simulink model "entryVehicle"  (R2024b)
settings: Solver=ode5  StartTime=startTime  StopTime=stopTime  FixedStep=stepTime  RelTol=1e-3
values from neighbouring files (symbols this model uses):
  acce_bias = [0; 0; 0]    [run_entryVehicle.m]
  acce_S = [0, 0, 0 ... (first row only)    [run_entryVehicle.m]
  alpha_0 = deg2rad(-23.82)    [run_entryVehicle.m]
  beta_0 = deg2rad(0.0)    [run_entryVehicle.m]
  chi_0 = deg2rad(90)    [run_entryVehicle.m]
  d_ref = 3.9    [run_entryVehicle.m]
  gamma_0 = deg2rad(-9.536)    [run_entryVehicle.m]
  H_s = 7050    [run_entryVehicle.m]
  I_xx = 5617.61    [run_entryVehicle.m]
  I_xz = 0    [run_entryVehicle.m]
  I_yy = 4454.62    [run_entryVehicle.m]
  I_zz = 4454.80    (= 4454.8)    [run_entryVehicle.m]
  lambda_0 = deg2rad(0)    [run_entryVehicle.m]
  m_0 = 4976    [run_entryVehicle.m]
  Mars_radius = 6371e3    (= 6371000)    [run_entryVehicle.m]
  p_0 = deg2rad(0)    [run_entryVehicle.m]
  Q0 = [Q1; Q2; Q3; Q4]    [get_Q0.m]    (also in run_entryVehicle.m = get_Q0(tau_0, lambda_0, chi_0, gamma_0, alpha_0, beta_0, sig)
  q_0 = deg2rad(0)    [run_entryVehicle.m]
  r0_eci = [x; y; z]    [getInitialECI.m]
  r_0 = deg2rad(0)    [run_entryVehicle.m]
  R_0 = 220e3 + Mars_radius    (= 6591000)    [run_entryVehicle.m]
  r_cm = [-0.137; 0; 1.8]    [run_entryVehicle.m]
  R_s = 287    [run_entryVehicle.m]
  rateGyro_bias = [0; 0; 0]    [run_entryVehicle.m]
  rateGyro_S = [0, 0, 0 ... (first row only)    [run_entryVehicle.m]
  rho_0 = 1.225    [run_entryVehicle.m]
  S_ref = 12    [run_entryVehicle.m]
  sigma_0 = deg2rad(100.)    [run_entryVehicle.m]
  specific_heat = 1.29    [run_entryVehicle.m]
  stepTime = 0.01    [run_entryVehicle.m]
  tau_0 = deg2rad(0)    [run_entryVehicle.m]
  v0_eci = T_ECI_NED * v_ned    [getInitialECI.m]
  V_0 = 11e3    (= 11000)    [run_entryVehicle.m]
undefined symbols (not defined in the file or in its folder): A_attitude, alpha_T_CD, alpha_T_CL, alpha_T_Cm, alpha_T_Cm_q, B_attitude, CD_T, CL_T, Cm_qT, Cm_T, K_lat, K_long, lateral_ref, longitudinal_ref, Mach_numbers_CD, Mach_numbers_CL, Mach_numbers_Cm, Mach_numbers_Cm_q, Mars_mu, my_max
libraries: simulink_extras x33, aerolibnav x2, simulink x1, SignalEditorBlockLib x1
(part 2 of 2)

== system entryVehicle/State Space/References ==
  lateral_ref : Constant  Value=lateral_ref
  longitudinal_ref : Constant  Value=longitudinal_ref
  out_longitudinal ref : Outport
  out_lateral_ref : Outport  Port=2
  wires:
  longitudinal_ref/1 -> out_longitudinal ref/1
  lateral_ref/1 -> out_lateral_ref/1

== system entryVehicle/Plant/Atmosphere/Atmospheric Density ==
  h : Inport
  Constant : Constant  Value=rho_0  SampleTime=stepTime
  Constant1 : Constant  Value=H_s  SampleTime=stepTime
  MATLAB Function : MATLAB Function  TreatAsAtomicUnit=on
  rho : Outport
  wires:
  h/1 -> MATLAB Function/1(h)
  Constant1/1 -> MATLAB Function/3(H_s)
  Constant/1 -> MATLAB Function/2(rho_0)
  MATLAB Function/1(rho) -> rho/1

== system entryVehicle/Plant/Dynamics/Attitude Dynamics ==
  M_x : Inport
  M_y : Inport  Port=2
  M_z : Inport  Port=3
  p : Inport  Port=4
  q : Inport  Port=5
  r : Inport  Port=6
  Ixx : Inport  Port=7
  Iyy : Inport  Port=8
  Izz : Inport  Port=9
  Ixz : Inport  Port=10
  Integrator : Integrator  InitialCondition=p_0
  Integrator1 : Integrator  InitialCondition=q_0
  Integrator2 : Integrator  InitialCondition=r_0
  MATLAB Function1 : MATLAB Function  TreatAsAtomicUnit=on
  Mux : Mux  Inputs=3
  p,q,r : Outport
  wires:
  MATLAB Function1/2(q_dot) -> Integrator1/1
  MATLAB Function1/1(p_dot) -> Integrator/1
  MATLAB Function1/3(r_dot) -> Integrator2/1
  Integrator/1 -> Mux/1  "p"
  Integrator1/1 -> Mux/2  "q"
  Integrator2/1 -> Mux/3  "r"
  Mux/1 -> p,q,r/1
  M_x/1 -> MATLAB Function1/1(M_x)
  M_y/1 -> MATLAB Function1/2(M_y)
  M_z/1 -> MATLAB Function1/3(M_z)
  p/1 -> MATLAB Function1/4(p)
  q/1 -> MATLAB Function1/5(q)
  r/1 -> MATLAB Function1/6(r)
  Ixx/1 -> MATLAB Function1/7(Ixx)
  Iyy/1 -> MATLAB Function1/8(Iyy)
  Izz/1 -> MATLAB Function1/9(Izz)
  Ixz/1 -> MATLAB Function1/10(Ixz)

== system entryVehicle/Plant/Dynamics/Heat_Flux ==
  rho : Inport
  V : Inport  Port=2
  MATLAB Function : MATLAB Function  TreatAsAtomicUnit=on
  To Workspace : ToWorkspace  VariableName=q_c  SaveFormat=Timeseries  SampleTime=-1
  q_c : Outport
  wires:
  rho/1 -> MATLAB Function/2(rho)
  V/1 -> MATLAB Function/1(V)
  MATLAB Function/1(q_c) -> To Workspace/1, q_c/1

== system entryVehicle/Plant/Dynamics/Translation Dynamics ==
  D : Inport
  L : Inport  Port=2
  S : Inport  Port=3
  V : Inport  Port=4
  gamma : Inport  Port=5
  chi : Inport  Port=6
  sigma : Inport  Port=7
  R : Inport  Port=8
  lambda : Inport  Port=9
  m : Inport  Port=10
  g : Inport  Port=11
  Integrator : Integrator  InitialCondition=V_0
  Integrator1 : Integrator  InitialCondition=gamma_0
  Integrator2 : Integrator  InitialCondition=chi_0
  MATLAB Function : MATLAB Function  TreatAsAtomicUnit=on
  Mux : Mux  Inputs=3
  V,gamma,chi : Outport
  wires:
  MATLAB Function/1(V_dot) -> Integrator/1
  MATLAB Function/2(gamma_dot) -> Integrator1/1
  MATLAB Function/3(chi_dot) -> Integrator2/1
  Integrator/1 -> Mux/1  "V"
  Integrator1/1 -> Mux/2  "gamma"
  Integrator2/1 -> Mux/3  "chi"
  Mux/1 -> V,gamma,chi/1
  D/1 -> MATLAB Function/1(D)
  L/1 -> MATLAB Function/2(L)
  S/1 -> MATLAB Function/3(S)
  V/1 -> MATLAB Function/4(V)
  gamma/1 -> MATLAB Function/5(gamma)
  chi/1 -> MATLAB Function/6(chi)
  sigma/1 -> MATLAB Function/7(sigma)
  R/1 -> MATLAB Function/8(R)
  lambda/1 -> MATLAB Function/9(lambda)
  m/1 -> MATLAB Function/10(m)
  g/1 -> MATLAB Function/11(g)

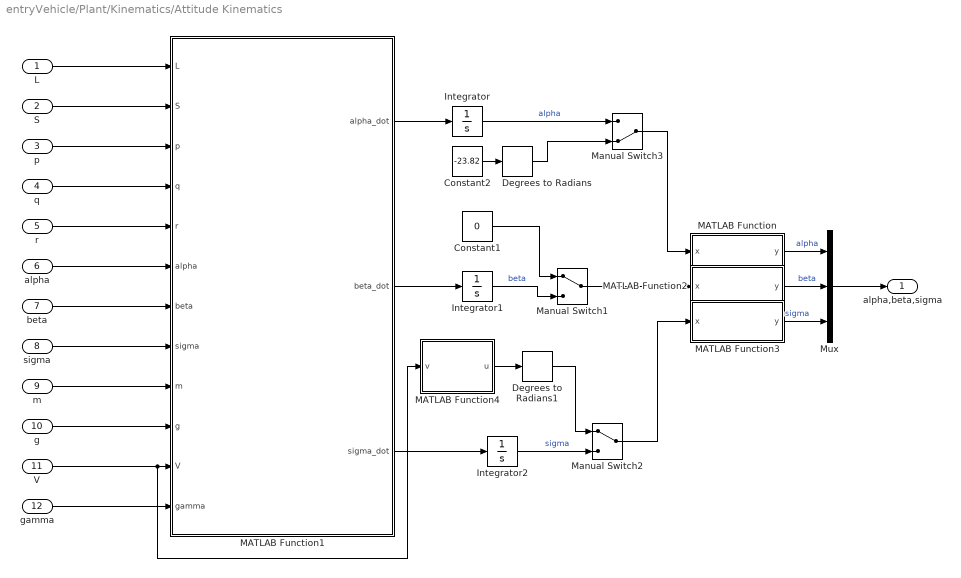
== system entryVehicle/Plant/Kinematics/Attitude Kinematics ==
  L : Inport
  S : Inport  Port=2
  p : Inport  Port=3
  q : Inport  Port=4
  r : Inport  Port=5
  alpha : Inport  Port=6
  beta : Inport  Port=7
  sigma : Inport  Port=8
  m : Inport  Port=9
  g : Inport  Port=10
  V : Inport  Port=11
  gamma : Inport  Port=12
  Constant1 : Constant  Value=0
  Constant2 : Constant  Value=-23.82
  Degrees to Radians : simulink_extras/Transformations/Degrees to Radians
  Degrees to Radians1 : simulink_extras/Transformations/Degrees to Radians
  Integrator : Integrator  InitialCondition=alpha_0
  Integrator1 : Integrator  InitialCondition=beta_0
  Integrator2 : Integrator  InitialCondition=sigma_0
  MATLAB Function : MATLAB Function  TreatAsAtomicUnit=on
  MATLAB Function1 : MATLAB Function  TreatAsAtomicUnit=on
  MATLAB Function2 : MATLAB Function  TreatAsAtomicUnit=on
  MATLAB Function3 : MATLAB Function  TreatAsAtomicUnit=on
  MATLAB Function4 : MATLAB Function  TreatAsAtomicUnit=on
  Manual Switch1 : ManualSwitch
  Manual Switch2 : ManualSwitch
  Manual Switch3 : ManualSwitch  CurrentSetting=0
  Mux : Mux  Inputs=3
  alpha,beta,sigma : Outport
  wires:
  beta/1 -> MATLAB Function1/7(beta)
  q/1 -> MATLAB Function1/4(q)
  m/1 -> MATLAB Function1/9(m)
  p/1 -> MATLAB Function1/3(p)
  sigma/1 -> MATLAB Function1/8(sigma)
  alpha/1 -> MATLAB Function1/6(alpha)
  L/1 -> MATLAB Function1/1(L)
  r/1 -> MATLAB Function1/5(r)
  g/1 -> MATLAB Function1/10(g)
  V/1 -> MATLAB Function4/1(v), MATLAB Function1/11(V)
  Mux/1 -> alpha,beta,sigma/1
  gamma/1 -> MATLAB Function1/12(gamma)
  MATLAB Function/1(y) -> Mux/1  "alpha"
  MATLAB Function2/1(y) -> Mux/2  "beta"
  MATLAB Function3/1(y) -> Mux/3  "sigma"
  S/1 -> MATLAB Function1/2(S)
  MATLAB Function1/1(alpha_dot) -> Integrator/1
  MATLAB Function1/2(beta_dot) -> Integrator1/1
  MATLAB Function1/3(sigma_dot) -> Integrator2/1
  Constant2/1 -> Degrees to Radians/1
  Integrator/1 -> Manual Switch3/1  "alpha"
  Manual Switch3/1 -> MATLAB Function/1(x)
  Manual Switch1/1 -> MATLAB Function2/1(x)
  Integrator1/1 -> Manual Switch1/2  "beta"
  Constant1/1 -> Manual Switch1/1
  Manual Switch2/1 -> MATLAB Function3/1(x)
  Integrator2/1 -> Manual Switch2/2  "sigma"
  Degrees to Radians/1 -> Manual Switch3/2
  Degrees to Radians1/1 -> Manual Switch2/1
  MATLAB Function4/1(u) -> Degrees to Radians1/1

== system entryVehicle/Plant/Kinematics/Translation Kinematics ==
  V : Inport
  gamma : Inport  Port=2
  chi : Inport  Port=3
  R : Inport  Port=4
  lambda : Inport  Port=5
  Integrator : Integrator  InitialCondition=R_0
  Integrator1 : Integrator  InitialCondition=tau_0
  Integrator2 : Integrator  InitialCondition=lambda_0
  MATLAB Function : MATLAB Function  TreatAsAtomicUnit=on
  Mux : Mux  Inputs=3
  R,tau,lambda : Outport
  wires:
  V/1 -> MATLAB Function/1(V)
  gamma/1 -> MATLAB Function/2(gamma)
  chi/1 -> MATLAB Function/3(chi)
  R/1 -> MATLAB Function/4(R)
  lambda/1 -> MATLAB Function/5(lambda)
  MATLAB Function/1(R_dot) -> Integrator/1
  MATLAB Function/2(tau_dot) -> Integrator1/1
  MATLAB Function/3(lambda_dot) -> Integrator2/1
  Integrator/1 -> Mux/1
  Integrator1/1 -> Mux/2
  Integrator2/1 -> Mux/3
  Mux/1 -> R,tau,lambda/1

== matlab function entryVehicle/Plant/Dynamics/Translation Dynamics/MATLAB Function ==
  data: V_dot output; gamma_dot output; chi_dot output; D input; L input; S input; V input; gamma input; chi input; sigma input; R input; lambda input; m input; g input
function [V_dot, gamma_dot, chi_dot] = Translation_Dynamics(D, L, S, V, gamma, chi, sigma, R, lambda, m, g)

V_dot = -D/m - g*sin(gamma);
gamma_dot = (V/R - g/V)*cos(gamma) + (L*cos(sigma) - S*sin(sigma))/(m*V);
chi_dot = V/R*cos(gamma)*tan(lambda)*sin(chi) - (L*sin(sigma) + S*cos(sigma))/(m*V*cos(gamma));

== matlab function entryVehicle/Plant/Aerodynamic Data (Apex reference frame)/MATLAB Function1 ==
  data: alpha input; alphaT output; beta input
function alphaT = total_angleAttack(alpha, beta)

alphaT = acos(cos(alpha)*cos(beta));

== matlab function entryVehicle/Plant/Aerodynamic Data (Apex reference frame)/MATLAB Function2 ==
  data: C_m output; C_mT input; C_n output; alpha input; beta input; alphaT input
function [C_m, C_n] = CmTtransformation(C_mT, alpha, beta, alphaT)

epsilon = 1e-6; % Threshold to detect near-zero total angle

if abs(alphaT) < epsilon
    % At singularity: alpha = beta = 0, so just return total coefficient for pitch moment, no yaw moment
    C_m = C_mT;
    C_n = 0;
else
    % Regular transformation
    C_m = sin(alpha)*cos(beta)/sin(alphaT) * C_mT;
    C_n = -sin(beta)/sin(alphaT) * C_mT;
end

== matlab function entryVehicle/Plant/Aerodynamic Data (Apex reference frame)/MATLAB Function3 ==
  data: C_mq output; C_mqT input; C_nr output; alpha input; beta input; alphaT input
function [C_mq, C_nr] = CmqTtransformation(C_mqT, alpha, beta, alphaT)

epsilon = 1e-6; % Threshold to detect near-zero total angle

if abs(alphaT) < epsilon
    % At singularity: alpha = beta = 0, so just return total coefficient for pitch moment, no yaw moment
    C_mq = C_mqT;
    C_nr = 0;
else
    % Regular transformation
    C_mq = sin(alpha)*cos(beta)/sin(alphaT) * C_mqT;
    C_nr = -sin(beta)/sin(alphaT) * C_mqT;
end

== matlab function entryVehicle/Plant/Kinematics/Attitude Kinematics/MATLAB Function ==
  data: x input; y output
function y = wrap_angle(x)
    y = wrapToPi(x);
end

== matlab function entryVehicle/Plant/Kinematics/Attitude Kinematics/MATLAB Function2 ==
  data: x input; y output
function y = wrap_angle(x)
    y = wrapToPi(x);
end

== matlab function entryVehicle/Plant/Kinematics/Attitude Kinematics/MATLAB Function3 ==
  data: x input; y output
function y = wrap_angle(x)
    y = wrapToPi(x);
end

== matlab function entryVehicle/Plant/Moments/MATLAB Function ==
  data: Mx_cross output; My_cross output; Mz_cross output; X_A input; Y_A input; Z_A input; r_cm input
function [Mx_cross, My_cross, Mz_cross] = crossProduct(X_A, Y_A, Z_A, r_cm)
    % Force vector in apex axes: [X; Y; Z]
    F_A_apex = [X_A; Y_A; Z_A];

    % Cross product to shift moment from apex to center of mass
    M_cross = cross(r_cm, F_A_apex);

    % Output individual components
    Mx_cross = M_cross(1);
    My_cross = M_cross(2);
    Mz_cross = M_cross(3);
end

== matlab function entryVehicle/Plant/Moments/MATLAB Function1 ==
  data: D input; X_A output; L input; S input; alpha input; beta input; Y_A output; Z_A output
function [X_A, Y_A, Z_A] = aeroFrame2apexFrameForces(D, L, S, alpha, beta)

c_alpha = cos(alpha);
s_alpha = sin(alpha);
c_beta = cos(beta);
s_beta = sin(beta);

X_A = -D*c_alpha*c_beta + S*c_alpha*s_beta + L*s_alpha;
Y_A = -D*s_beta - S*c_beta;
Z_A = -D*s_alpha*c_beta + S*s_alpha*s_beta - L*c_alpha;

== matlab function entryVehicle/State Space/MATLAB Function ==
  data: My input; u output; Mtx_Mtz input
function u = combine(My, Mtx_Mtz)
    Mx = Mtx_Mtz(1);
    Mz = Mtx_Mtz(2);
    
    u = [Mx; My; Mz];
end

== matlab function entryVehicle/Controller/Lateral Gain Scheduling/MATLAB Function ==
  data: Mach input; K_lat output
function K_lat = getLateralGain(Mach)
%#codegen
persistent Mach_Klat K_lat_data

if isempty(Mach_Klat)
    S = load('KLateralLUT.mat');  % Loads [N x 8]
    Mach_Klat = S.Mach_Klat;
    K_lat_data = S.K_lat_data;  % N x 8 (flattened 2x4)
end

% Interpolate 8 gains
K_lat_flat = interp1(Mach_Klat, K_lat_data, Mach, 'linear', 'extrap');

% Reshape into 2x4 matrix
K_lat = reshape(K_lat_flat, [2, 4]);
end

== matlab function entryVehicle/Controller/Longitude Gain Scheduling/MATLAB Function ==
  data: Mach input; K_long output
function K_long = getLongitudinalGain(Mach)
%#codegen
persistent Mach_Klong K_long_data

if isempty(Mach_Klong)
    S = load('KLongitudinalLUT.mat');  % <-- Load into struct first
    Mach_Klong = S.Mach_Klong;
    K_long_data = S.K_long_data;
end

% Interpolate both gains
K_long1 = interp1(Mach_Klong, K_long_data, Mach, 'linear', 'extrap');  % returns 1x2 vector
K_long = K_long1.';  % Now it's [2x1]
end

== matlab function entryVehicle/Controller/Integrator Subsystem/MATLAB Function ==
  data: Mach input; K_integrator_sigma output
function K_integrator_sigma = getIntsigmaGain(Mach)
%#codegen
persistent Mach_Ksigma K_sigmaInt_data

if isempty(Mach_Ksigma)
    S = load('KsigmaIntLUT.mat');  % Loads gain schedule
    Mach_Ksigma = S.Mach_Ksigma;          % Breakpoints
    K_sigmaInt_data = S.K_sigmaInt_data;  % Scalar gains
end

% Interpolate scalar gain based on Mach
K_integrator_sigma = interp1(Mach_Ksigma, K_sigmaInt_data, Mach, 'linear', 'extrap');
end

== matlab function entryVehicle/Controller/Integrator Subsystem1/MATLAB Function ==
  data: Mach input; K_integrator_alpha output
function K_integrator_alpha= getIntalphaGain(Mach)
%#codegen
persistent Mach_Ksigma K_sigmaInt_data

if isempty(Mach_Ksigma)
    S = load('KsigmaIntLUT.mat');  % Loads gain schedule
    Mach_Ksigma = S.Mach_Ksigma;          % Breakpoints
    K_sigmaInt_data = S.K_sigmaInt_data;  % Scalar gains
end

% Interpolate scalar gain based on Mach
K_integrator_alpha = interp1(Mach_Ksigma, K_sigmaInt_data, Mach, 'linear', 'extrap');
end

== matlab function entryVehicle/Plant/Kinematics/Attitude Kinematics/MATLAB Function4 ==
  data: v input; u output
function u = reference(v)

if v >= 3500
    u = 100;
elseif v <= 1500
    u = 75;
else
    u = 75 + (100 - 75) * (v - 1500) / (3500 - 1500);
end

== matlab function entryVehicle/Plant/Dynamics/Heat_Flux/MATLAB Function ==
  data: V input; q_c output; rho input
function q_c = heatFluxChapman(V, rho)
%#codegen

% Constants
c1 = 1.83e-4;     % empirical constant [SI]
c2 = 3.0;   % velocity exponent
d_ref = 3.9;
Rn = d_ref;         % nose radius [m]

% Chapman cold-wall heat flux equation
q_c = c1 / sqrt(Rn) * sqrt(rho) * V^c2;
end

== matlab function entryVehicle/Navigation/IMU Sensor2/MATLAB Function ==
  data: g_vec output; r input
function g_vec = computegvec(r)
% r    : 3x1 position vector in ECI frame (m)
% Constants
mu = 3.98319648e14; % Earth's gravitational parameter (m^3/s^2)

% Compute gravity vector in inertial frame
r_norm = norm(r);
g_vec1 = -mu / r_norm^3 * r;
g_vec=g_vec1';
end

== matlab function entryVehicle/Guidance/MATLAB Function ==
  data: x input; h output; s_dot output; m input; S_ref input; beta input; L_D input; rho_0 input; H_s input; v_dot output; L_D output; m output; gamma_dot output; h_dot output; D output
function [h,s_dot, v_dot, L_D, m, gamma_dot, h_dot, D] = entry_dynamics_derivatives(x, m, S_ref, beta, L_D, rho_0, H_s)
% Computes simplified translational dynamics for entry guidance
%
% Inputs:
%   x      : state vector [R; tau; delta; alpha; beta; sigma; v; gamma; chi; p; q; r]
%   m      : vehicle mass [kg]
%   S_ref  : reference area [m^2]
%   beta   : ballistic coefficient [kg/m^2]
%   L_D    : lift-to-drag ratio
%   rho_0  : reference atmospheric density [kg/m^3]
%   H_s    : scale height of the atmosphere [m]
%
% Output:
%   x_dot  : [s_dot; v_dot; gamma_dot; h_dot]

% ==== 1. Unpack necessary state variables ====
Mars_radius = 6371e3;
R     = x(1);   % Radius [m]
h = R-Mars_radius;
sigma = x(6);   % Bank angle [rad]
v     = x(7);   % Velocity [m/s]
gamma = x(8);   % Flight path angle [rad]

% ==== 2. Constants ====
Re = 6371e3;         % Earth radius [m]
g0 = 9.80665;        % Gravity at sea level [m/s^2]
h  = R - Re;         % Altitude [m]
gs = g0 * (Re / R)^2;  % Local gravity at R

% ==== 3. Atmospheric density ====
rho = rho_0 * exp(-h / H_s);

% ==== 4. Drag and Lift ====
C_D = m / (beta * S_ref);                      % Drag coefficient
D   = 0.5 * rho * v^2 * C_D * S_ref;           % Drag force [N]
L   = L_D * D;                                 % Lift force [N]

% ==== 5. Equations ====
s_dot     = v * cos(gamma);                                % Range rate
v_dot     = - (D/m + gs * sin(gamma));                     % Velocity rate
gamma_dot = (L * cos(sigma)) / (m * v) + ...
            ((v / R) - (gs / v)) * cos(gamma);             % Flight path angle rate
h_dot     = v * sin(gamma);                                % Altitude rate
end

== matlab function entryVehicle/Navigation/IMU Sensor3/MATLAB Function ==
  data: g_vec output; r input
function g_vec = computegvec(r)
% r    : 3x1 position vector in ECI frame (m)
% Constants
mu = 3.98319648e14; % Earth's gravitational parameter (m^3/s^2)

% Compute gravity vector in inertial frame
r_norm = norm(r);
g_vec1 = -mu / r_norm^3 * r;
g_vec=g_vec1';
end

== matlab function entryVehicle/Navigation/IMU Sensor3/MATLAB Function6 ==
  data: Q input; omega input; Q_dot output
function Q_dot = quat_kinematics(Q, omega)
    % omega: 3x1 vector [wx; wy; wz]
    % Q: 4x1 quaternion [q1; q2; q3; q4] (q4 is scalar part)
    Omega = [     0   -omega(1) -omega(2) -omega(3);
               omega(1)     0    omega(3) -omega(2);
               omega(2) -omega(3)     0    omega(1);
               omega(3)  omega(2) -omega(1)     0   ];
    Q_dot = 0.5 * Omega * Q;
end

== matlab function entryVehicle/Navigation/IMU Sensor3/MATLAB Function7 ==
  data: Q input; TIC output
function TIC = quatToDCM(Q)
% Q = [q1; q2; q3; q4]  (q4 is scalar part)

q1 = Q(1); q2 = Q(2); q3 = Q(3); q4 = Q(4);
TIC = [1 - 2*(q2^2 + q3^2),     2*(q1*q2 + q3*q4),     2*(q1*q3 - q2*q4);
     2*(q1*q2 - q3*q4),       1 - 2*(q1^2 + q3^2),   2*(q2*q3 + q1*q4);
     2*(q1*q3 + q2*q4),       2*(q2*q3 - q1*q4),     1 - 2*(q1^2 + q2^2)];
end

== matlab function entryVehicle/Navigation/State to Body (acce minus gravity)/MATLAB Function3 ==
  data: alpha_beta_sigma input; V_gamma_chi input; g_b output; R_tau_delta input; mu input
function g_b = computeGravityBody(alpha_beta_sigma, V_gamma_chi, R_tau_delta, mu)
    
    alpha = alpha_beta_sigma(1);
    beta = alpha_beta_sigma(2);
    sigma = alpha_beta_sigma(3);

    gamma = V_gamma_chi(2);
    chi = V_gamma_chi(3);

    R = R_tau_delta(1);

    % Gravity in vertical frame (downward)
    g_v = [0; 0; mu / R^2];

    % Precompute trigonometric values
    cchi = cos(chi);
    schi = sin(chi);
    cgamma = cos(gamma);
    sgamma = sin(gamma);
    calpha = cos(alpha);
    salpha = sin(alpha);
    cbeta = cos(beta);
    sbeta = sin(beta);
    csigma = cos(sigma);
    ssigma = sin(sigma);

    % Rotation from aerodynamic to vertical
    R_v_aa = [ ...
        cchi*cgamma, -schi*csigma - cchi*sgamma*ssigma, -schi*ssigma + cchi*sgamma*csigma;
        schi*cgamma,  cchi*csigma - schi*sgamma*ssigma,  cchi*sgamma + schi*sgamma*csigma;
       -sgamma,      -cgamma*ssigma,                    cgamma*csigma ...
    ];

    R_aa_v = R_v_aa';

    % Rotation from body to aerodynamic
    R_aa_b = [ ...
        calpha*cbeta,  sbeta,         salpha*cbeta;
       -calpha*sbeta,  cbeta,        -salpha*sbeta;
       -salpha,        0,             calpha ...
    ];

    R_b_aa = R_aa_b';

    % Rotate gravity into body frame
    g_b = R_b_aa * R_aa_v * g_v;
end

== matlab function entryVehicle/Navigation/State to Body (acce minus gravity)/MATLAB Function4 ==
  data: alpha_beta_sigma input; V_gamma_chi input; u_v_w output
function u_v_w = computeV_body(alpha_beta_sigma, V_gamma_chi)
% computeV_body calculates the velocity vector in the body frame (u, v, w)
% given aerodynamic angles (alpha, beta) and inertial flight conditions.
%
% Inputs:
%   alpha_beta_sigma : [alpha; beta; sigma] in radians
%       - alpha : angle of attack (pitch angle of velocity vector)
%       - beta  : sideslip angle (lateral deviation of velocity vector)
%
%   V_gamma_chi : [V; gamma; chi]
%       - V     : total airspeed (or speed over ground)
%
% Output:
%   u_v_w : [u; v; w] velocity components in body frame
%       - u: forward velocity (along x-axis)
%       - v: lateral velocity (along y-axis)
%       - w: vertical velocity (along z-axis)

% Extract total speed
V = V_gamma_chi(1);

% Extract aerodynamic angles
alpha = alpha_beta_sigma(1);  % angle of attack
beta  = alpha_beta_sigma(2);  % sideslip angle

% Compute body-frame velocity components using standard aero kinematics
u = V * cos(alpha) * cos(beta);  % forward component
v = V * sin(beta);               % lateral (side-slip) component
w = V * sin(alpha) * cos(beta);  % vertical component

% Return as a column vector
u_v_w = [u; v; w];

end

== matlab function entryVehicle/Guidance/MATLAB Function3 ==
  data: s_dot input; s output; h input; sample_time input
function s = integrate_s_dot(s_dot, h, sample_time)
    persistent s_prev s_dot_prev

    if isempty(s_prev)
        s_prev = 0;
    end
    if isempty(s_dot_prev)
        s_dot_prev = s_dot;
    end

    dt = sample_time;

    if h ~= 0
        % Trapézio: usa valor atual e anterior
        s_prev = s_prev + 0.5 * dt * (s_dot + s_dot_prev);
    end

    s = s_prev;
    s_dot_prev = s_dot;  % Atualizar para o próximo passo
end

== matlab function entryVehicle/Navigation/MATLAB Function ==
  data: u input; y output
function y = fcn(u)

y = norm(u);

== matlab function entryVehicle/Navigation/MATLAB Function1 ==
  data: u input; y output
function y = fcn(u)

y = norm(u);

== matlab function entryVehicle/Navigation/ECI State to State/MATLAB Function3 ==
  data: Q input; alpha_beta_sigma output; V_gamma_chi input; R_tau_delta input
function alpha_beta_sigma = quat2aeroAngles(Q, V_gamma_chi, R_tau_delta)
% Inputs:
% Q            : 4x1 quaternion [q1; q2; q3; q4] (scalar last)
% V_gamma_chi  : [V; gamma; chi]
% R_tau_lambda : [r; tau; lambda] -> tau: latitude, lambda: longitude

% Extract quaternion elements
q1 = Q(1); q2 = Q(2); q3 = Q(3); q4 = Q(4);

% Direction cosine matrix from body to inertial frame
C_IB = [ ...
    q1^2 + q4^2 - q2^2 - q3^2,   2*(q1*q2 + q3*q4),       2*(q1*q3 - q2*q4);
    2*(q1*q2 - q3*q4),           q2^2 + q4^2 - q1^2 - q3^2, 2*(q2*q3 + q1*q4);
    2*(q1*q3 + q2*q4),           2*(q2*q3 - q1*q4),       q3^2 + q4^2 - q1^2 - q2^2 ...
];

% Extract trajectory angles
gamma = V_gamma_chi(2);  % flight path angle
chi   = V_gamma_chi(3);  % heading angle

% Extract latitude and longitude
tau = R_tau_delta(2);   % latitude
delta = R_tau_delta(3);% longitude

% C_TV = C2(gamma) * C3(chi)
cgamma = cos(gamma);
sgamma = sin(gamma);
cchi = cos(chi);
schi = sin(chi);
C_TV = [cgamma*cchi,  schi*cgamma,  -sgamma;
       -schi,     cchi,      0;
        cchi*sgamma,  schi*sgamma,   cgamma];

% C_VI = C2(-delta - pi/2) * C3(tau)
cdelta = cos(delta);
sdelta = sin(delta);
ct = cos(tau);
st = sin(tau);

C_VI = [ ...
    -ct*sdelta,  -st*sdelta,  cdelta;
    -st,      ct,     0;
    -ct*cdelta,  -st*cdelta, -sdelta
];

% Compose full transformation: C_TB
C_TB = C_TV * C_VI * C_IB;

% Extract angles
alpha  = atan2(C_TB(1,3), C_TB(1,1));   % [rad]
beta   = asin(C_TB(1,2));               % [rad]
sigma  = atan2(-C_TB(3,2), C_TB(2,2));  % [rad]

% Output
alpha_beta_sigma = [alpha; beta; sigma];
end

== matlab function entryVehicle/Navigation/IMU Sensor/MATLAB Function1 ==
  data: omega_true input; omega_measured output; b_gyro input; S_omega input
function omega_measured = gyroModel(omega_true, b_gyro, S_omega)
% omega_true     : true angular velocity [3x1]
% b_gyro         : gyroscope bias vector [3x1]
% S_omega        : scale factor + misalignment matrix [3x3]
% omega_measured : measured angular velocity [3x1]

%#codegen

% Identity matrix
I3 = eye(3);

% Measurement model: ω_m = b_ω + (I + S_ω) * ω
omega_measured = b_gyro + (I3 + S_omega) * omega_true;

end

== matlab function entryVehicle/Navigation/IMU Sensor2/MATLAB Function6 ==
  data: Q input; omega input; Q_dot output
function Q_dot = quat_kinematics(Q, omega)
    % omega: 3x1 vector [wx; wy; wz]
    % Q: 4x1 quaternion [q1; q2; q3; q4] (q4 is scalar part)
    Omega = [     0   -omega(1) -omega(2) -omega(3);
               omega(1)     0    omega(3) -omega(2);
               omega(2) -omega(3)     0    omega(1);
               omega(3)  omega(2) -omega(1)     0   ];
    Q_dot = 0.5 * Omega * Q;
end

== matlab function entryVehicle/Navigation/IMU Sensor2/MATLAB Function7 ==
  data: Q input; TIC output
function TIC = quatToDCM(Q)
% Q = [q1; q2; q3; q4]  (q4 is scalar part)

q1 = Q(1); q2 = Q(2); q3 = Q(3); q4 = Q(4);
TIC = [1 - 2*(q2^2 + q3^2),     2*(q1*q2 + q3*q4),     2*(q1*q3 - q2*q4);
     2*(q1*q2 - q3*q4),       1 - 2*(q1^2 + q3^2),   2*(q2*q3 + q1*q4);
     2*(q1*q3 + q2*q4),       2*(q2*q3 - q1*q4),     1 - 2*(q1^2 + q2^2)];
end

== matlab function entryVehicle/User Commands/MATLAB Function ==
  data: v input; u output
function u = reference(v)

if v >= 3500
    u = 100;
elseif v <= 1500
    u = 75;
else
    u = 75 + (100 - 75) * (v - 1500) / (3500 - 1500);
end

== matlab function entryVehicle/Guidance/MATLAB Function2 ==
  data: s input; s_star input; hdot input; hdot_star input; D input; D_star input; L_D input; m input; phi_cmd output; F1 input; F2 input; F3 input; sigma_star input; v input; u1 output; delta_s output; delta_hdot output; delta_Doverm output
function [phi_cmd, u1, delta_s, delta_hdot, delta_Doverm] = apolloBankControlLaw( ...
    s, s_star, hdot, hdot_star, D, D_star, L_D, m, F1, F2, F3, sigma_star, v)

% Overcontrol factor
K = 5;

% Initialize outputs
u1 = 0;
delta_s = 0;
delta_hdot = 0;
delta_Doverm = 0;

% Select command based on velocity range
if v < 1000
    phi_cmd = deg2rad(75);  % Fixed low-speed command
elseif v > 10000
    phi_cmd = deg2rad(100);  % Fixed high-speed command
else
    % Control error terms
    delta_s = (s - s_star);
    delta_hdot = hdot - hdot_star;
    delta_Doverm = (D - D_star) / m;

    % Compute control command
    cossigma_star = cos(sigma_star);
    u = (5 / (F3)) * (-(delta_s) - F2 * delta_hdot + (F1) * delta_Doverm) + L_D*cossigma_star;
    u1 = u - L_D*cossigma_star;
    up = u/L_D;

    % Saturate and compute commanded bank angle
    up = max(min(up, 1), -1);
    phi_cmd = acos(up);
end

== matlab function entryVehicle/Guidance/MATLAB Function1 ==
  data: x input; F1 output; F2 output; F3 output; hdot_star output; s_star output; D_star output; sigma_star output; v output
function [F1, F2, F3, hdot_star, s_star, D_star, sigma_star,v] = getGuidanceReferenceValues(x)

v = x(7);   % Velocity [m/s]

% === Load persistent data once ===
persistent v_table F1_table F2_table F3_table hdot_table s_table D_table
if isempty(v_table)

    data = load('guidance_lookup_tables.mat');
    
    v_table     = data.v_unique_ds;
    hdot_table  = data.hdot_lut_ds;
    s_table     = data.s_lut_ds;
    D_table     = data.drag_lut_ds;
              length(D_table)
    F1_table = data.gain_table_ds.F1;
    F2_table = data.gain_table_ds.F2;
    F3_table = data.gain_table_ds.F3;
end


% === Interpolated values from lookup tables ===
F1         = interp1(v_table, F1_table, v, 'linear', 'extrap');
F2         = interp1(v_table, F2_table, v, 'linear', 'extrap');
F3         = interp1(v_table, F3_table, v, 'linear', 'extrap');
F3 = max(F3, 1e-4);
hdot_star  = interp1(v_table, hdot_table, v, 'linear', 'extrap');
s_star     = interp1(v_table, s_table, v, 'linear', 'extrap');
D_star     = interp1(v_table, D_table, v, 'linear', 'extrap');

% === Compute sigma_star from reference bank angle schedule ===
if v >= 3500
    sigma_star = deg2rad(100);
elseif v <= 1500
    sigma_star = deg2rad(75);
else
    sigma_star = deg2rad(75 + (100 - 75) * (v - 1500) / (3500 - 1500));
end

== matlab function entryVehicle/Navigation/ECI State to State/MATLAB Function ==
  data: r_ECI input; R_tau_delta output
function R_tau_delta = positionECI2spherical(r_ECI)

rx = r_ECI(1);
ry = r_ECI(2);
rz = r_ECI(3);

R = norm(r_ECI);
tau = atan2(ry,rx);
delta = asin(rz/R);

R_tau_delta = [R; tau; delta];

== matlab function entryVehicle/Navigation/ECI State to State/MATLAB Function1 ==
  data: v_ECI input; V_gamma_chi output; R_tau_delta input
function V_gamma_chi = velocityECI2trajectory(v_ECI, R_tau_delta)
% velocityECI2trajectory: Converts ECI velocity vector to flight-path variables
%
% Inputs:
%   v_ECI         - 3x1 velocity vector in ECI frame [vx; vy; vz]
%   R_tau_delta  - 3x1 position vector where:
%                     R_tau_delta(2) = tau   (heading angle, radians)
%                     R_tau_delta(3) = delta (flight path angle, radians)
%
% Output:
%   V_gamma_chi   - 3x1 vector: [V; chi; gamma]
%                     V     = speed magnitude
%                     gamma = flight path angle (elevation)
%                     chi   = azimuth angle (heading in horizontal plane)

% Extract angles from input
tau = R_tau_delta(2);    % Heading angle (chi), in radians
delta = R_tau_delta(3);  % Flight path angle (gamma), in radians

% Precompute trigonometric values for efficiency
ct = cos(tau);
st = sin(tau);
cd = cos(delta);
sd = sin(delta);

% Rotation matrix from vertical frame to ECI (or ECEF/ECI here assumed same)
% This transforms a vector from the local trajectory frame (velocity-based)
% into the inertial frame. Therefore, to go the other way, we transpose it.
C = [ -ct*sd,   -st,   -ct*cd;
      -st*sd,    ct,   -st*cd;
       cd,       0,    -sd ];

% Transform ECI velocity into vertical (trajectory-based) frame
v_Vertical = C' * v_ECI;

% Extract components in trajectory frame
vx = v_Vertical(1);  % Along velocity vector (forward)
vy = v_Vertical(2);  % Cross-track (horizontal right)
vz = v_Vertical(3);  % Vertical (upward)

% Compute magnitude of velocity
V = norm(v_ECI);

% Compute azimuth (heading angle) from velocity projection in local horizontal plane
chi = atan2(vy , vx);  % This is tan(chi), but may need atan2 for full quadrant info

% Compute flight path angle from vertical component
gamma = atan2(-vz , sqrt(vx^2 + vy^2));  % sin(gamma) = -vz / horizontal speed

% Pack output
V_gamma_chi = [V; gamma; chi];
end

== matlab function entryVehicle/Plant/Aerodynamic Data (Apex reference frame)/MATLAB Function ==
  data: C_L output; C_LT input; C_S output; alpha input; beta input; alphaT input
function [C_L, C_S] = CLTtransformation(C_LT, alpha, beta, alphaT)

epsilon = 1e-6; % Threshold to detect near-zero total angle

if abs(alphaT) < epsilon
    % At singularity: alpha = beta = 0, so just return total coefficient for lift, no sideforce
    C_L = C_LT;
    C_S = 0;
else
    % Regular transformation
    C_S = cos(alpha)*sin(beta)/sin(alphaT) * C_LT;
    C_L = sin(alpha)/sin(alphaT) * C_LT;
end

== matlab function entryVehicle/Navigation/ECI State to State/MATLAB Function2 ==
  data: u input; y output
function y = fcn(u)

y = norm(u);

== matlab function entryVehicle/Navigation/ECI State Propagation/MATLAB Function1 ==
  data: Q input; TIC output
function TIC = quatToDCM(Q)
% Q = [q1; q2; q3; q4]  (q4 is scalar part)

q1 = Q(1); q2 = Q(2); q3 = Q(3); q4 = Q(4);
TIC = [1 - 2*(q2^2 + q3^2),     2*(q1*q2 + q3*q4),     2*(q1*q3 - q2*q4);
     2*(q1*q2 - q3*q4),       1 - 2*(q1^2 + q3^2),   2*(q2*q3 + q1*q4);
     2*(q1*q3 + q2*q4),       2*(q2*q3 - q1*q4),     1 - 2*(q1^2 + q2^2)];
end

== matlab function entryVehicle/Navigation/ECI State Propagation/MATLAB Function2 ==
  data: Q input; omega input; Q_dot output
function Q_dot = quat_dynamics(Q, omega)
% Q: 4x1 quaternion (q1, q2, q3, q4), scalar last
% omega: 3x1 angular velocity vector [wx; wy; wz]

wx = omega(1);
wy = omega(2);
wz = omega(3);

% B matrix for quaternion derivative
B = [  0,   wz,  -wy,  wx;
      -wz,   0,   wx,  wy;
       wy, -wx,   0,   wz;
      -wx, -wy, -wz,   0 ];

Q_dot = 0.5 * B * Q;
end

== matlab function entryVehicle/Navigation/ECI State Propagation/MATLAB Function3 ==
  data: g_vec_ECI output; r_ECI input; mu input
function g_vec_ECI = computegvec(r_ECI, mu)
% r    : 3x1 position vector in ECI frame (m)
% mu

% Compute gravity vector in inertial frame
r_norm = norm(r_ECI);
g_vec_ECI = -mu / r_norm^3 * r_ECI;
end

== matlab function entryVehicle/Navigation/IMU Sensor/MATLAB Function ==
  data: a_body input; a_measured output; b_a input; S_a input
function a_measured = acceModel(a_body, b_a, S_a)
% a_body    : true specific force [3x1]
% b_a       : accelerometer bias vector [3x1]
% S_a       : scale+misalignment matrix [3x3]
% a_measured: measured acceleration minus gravity, in body frame [3x1]

%#codegen

% Identity matrix
I3 = eye(3);

% Measured acceleration according to: a_m = b + (I + Sa) * a_body
a_measured = b_a + (I3 + S_a) * a_body;

end

== matlab function entryVehicle/Navigation/State to Body (acce minus gravity)/MATLAB Function1 ==
  data: u input; y output
function y = fcn(u)

y = norm(u);

== matlab function entryVehicle/Navigation/State to Body (acce minus gravity)/MATLAB Function2 ==
  data: u input; y output
function y = fcn(u)

y = norm(u);

== matlab function entryVehicle/Navigation/State to Body (acce minus gravity)/MATLAB Function5 ==
  data: u input; y output
function y = fcn(u)

y = norm(u);

== matlab function entryVehicle/Navigation/State to Body (acce minus gravity)/MATLAB Function6 ==
  data: u input; y output
function y = fcn(u)

y = norm(u);

== matlab function entryVehicle/Navigation/ECI State Propagation/MATLAB Function ==
  data: Q_in input; Q_out output
function Q_out = normalizeQuat(Q_in)
    Q_out = Q_in / norm(Q_in);
end

== matlab function entryVehicle/Navigation/State to Body (acce minus gravity)/MATLAB Function ==
  data: alpha_beta_sigma input; Q0 output; R_tau_delta input; V_gamma_chi input
function Q0 = get_Q0(alpha_beta_sigma, R_tau_delta, V_gamma_chi)

    alpha_0 = alpha_beta_sigma(1);
    beta_0 = alpha_beta_sigma(2);
    sigma_0 = alpha_beta_sigma(3);

    gamma_0 = V_gamma_chi(2);
    chi_0 = V_gamma_chi(3);

    tau_0 = R_tau_delta(2);
    lambda_0 = R_tau_delta(3);
   
    % Precompute sines and cosines
    ct = cos(tau_0);
    st = sin(tau_0);
    cd = cos(lambda_0);
    sd = sin(lambda_0);
    
    cx = cos(chi_0);
    sx = sin(chi_0);
    cg = cos(gamma_0);
    sg = sin(gamma_0);
    
    cs = cos(sigma_0);
    ss = sin(sigma_0);
    cb = cos(beta_0);
    sb = sin(beta_0);
    ca = cos(alpha_0);
    sa = sin(alpha_0);
    
    % Matrix C_I,V
    C_IV = [ -ct*sd,      -st,   -ct*cd;
             -st*sd,       ct,   -st*cd;
                 cd,        0,       -sd ];
    
    % Matrix C_V,T
    C_VT = [ cx*cg,     -sx,   cx*sg;
             sx*cg,      cx,   sx*sg;
               -sg,       0,      cg ];
    
    % Matrix C_T,B
    C_TB = [ ca*cb,         sb,               sa*cb;
            -ca*sb*cs - sa*ss, cb*cs, ca*ss - sa*sb*cs;
             ca*sb*ss - sa*cs, -cb*ss, ca*cs + sa*sb*ss ];

    C_IB = C_IV * C_VT * C_TB;
    
    % Compute Q4 first
    Q4 = 0.5 * sqrt(1 + C_IB(1,1) + C_IB(2,2) + C_IB(3,3));
    
    % Compute Q1, Q2, Q3 based on Q4
    Q1 = (C_IB(2,3) - C_IB(3,2)) / (4 * Q4);
    Q2 = (C_IB(3,1) - C_IB(1,3)) / (4 * Q4);
    Q3 = (C_IB(1,2) - C_IB(2,1)) / (4 * Q4);
    
    % Quaternion as a column vector (or row vector if preferred)
    Q0 = [Q1; Q2; Q3; Q4];
    Q0 = Q0/norm(Q0);
end

== matlab function entryVehicle/Plant/Atmosphere/Atmospheric Density/MATLAB Function ==
  data: rho output; h input; rho_0 input; H_s input
function rho = Density(h, rho_0, H_s)

rho = rho_0 * exp(-h/H_s);

== matlab function entryVehicle/Plant/Kinematics/Translation Kinematics/MATLAB Function ==
  data: R_dot output; tau_dot output; lambda_dot output; V input; gamma input; chi input; R input; lambda input
function [R_dot, tau_dot, lambda_dot] = Translation_Kinematics(V, gamma, chi, R, lambda)

R_dot = V * sin(gamma);
tau_dot = (V * cos(gamma) * sin(chi)) / (R * cos(lambda));
lambda_dot = V / R * cos(gamma) * cos(chi);

== matlab function entryVehicle/Plant/Kinematics/Attitude Kinematics/MATLAB Function1 ==
  data: L input; S input; p input; q input; alpha_dot output; beta_dot output; sigma_dot output; r input; alpha input; beta input; sigma input; m input; g input; V input; gamma input
function [alpha_dot, beta_dot, sigma_dot] = Attitude_Kinematics(L, S, p, q, r, alpha, beta, sigma, m, g, V, gamma)

alpha_dot = q - (p*cos(alpha) + r*sin(alpha))*tan(beta) - (L - m*g*cos(gamma)*cos(sigma))/(m*V*cos(beta));
%alpha_dot = q - (p*cos(alpha) + r*sin(alpha))*tan(beta);
beta_dot = p*sin(alpha) - r*cos(alpha) - (S + m*g*cos(gamma)*sin(sigma))/(m*V);
%beta_dot = p*sin(alpha) - r*cos(alpha);
sigma_dot = -(p*cos(alpha) + r*sin(alpha))/(cos(beta)) - (L - m*g*cos(gamma)*cos(sigma))/(m*V)*tan(beta) + (L*sin(sigma) + S*cos(sigma))/(m*V)*tan(gamma);
%sigma_dot = -(p*cos(alpha) + r*sin(alpha))/(cos(beta));

if ~isfinite(alpha_dot)
    disp('Non-finite alpha_dot at t=0');
end

if any(~isfinite([L, S, p, q, r, alpha, beta, sigma, m, g, V, gamma]))
    disp('Invalid input at t=0:');
    disp([L, S, p, q, r, alpha, beta, sigma, m, g, V, gamma]);
end

== matlab function entryVehicle/Plant/Dynamics/Attitude Dynamics/MATLAB Function1 ==
  data: p_dot output; q_dot output; r_dot output; M_x input; M_y input; M_z input; p input; q input; r input; Ixx input; Iyy input; Izz input; Ixz input
function [p_dot, q_dot, r_dot] = Attitude_Dynamics(M_x, M_y, M_z, p, q, r, Ixx, Iyy, Izz, Ixz)

I_star = Ixx*Izz - Ixz*Ixz;

p_dot = Izz/I_star*M_x + Ixz/I_star*M_z + (Ixx-Iyy+Izz)*Ixz/I_star*p*q + ((Iyy-Izz)*Izz-Ixz^2)/I_star*q*r;
q_dot = M_y/Iyy + Ixz/Iyy*(r^2-p^2) + (Izz-Ixx)/Iyy*p*r;
r_dot = Ixz/I_star*M_x + Ixx/I_star*M_z + ((Ixx-Iyy)*Ixx + Ixz^2)/I_star*p*q + (-Ixx + Iyy - Izz)*Ixz/I_star*q*r;
